simulink model "chap5_5sim"  (Simulink 5.0)
settings: Solver=ode45  StartTime=0.0  StopTime=5.0  FixedStep=0.001  RelTol=1e-3
PreLoadFcn:
  | i=k;
settings Model: LastModifiedBy=Administrator  MaxDataPoints=10000  RTWOptions="-aEnforceIntegerDowncast=1 -aExtMode=0 -aExtModeTesting=0 -aFoldNonRolledExpr=1 -aForceParamTrailComments=0 -aGenerateComments=1 -aGenerateReport=0 -aIgnoreCustomStorageClasses=1 -aIncDataTypeInIds=0 -aIncHierarchyInIds=0 -aInlineInvariantSignals=0 -aInlinedPrmAccess=\"Literals\" -aLocalBlockOutputs=1 -aLogVarNameModifier=\"rt_\" -aMaxRTWIdLen=31 -aPrefixModelToSubsysFcnNames=1 -aRTWVerbose=1 -aRollThreshold=5 -aShowEliminatedStatements=0"

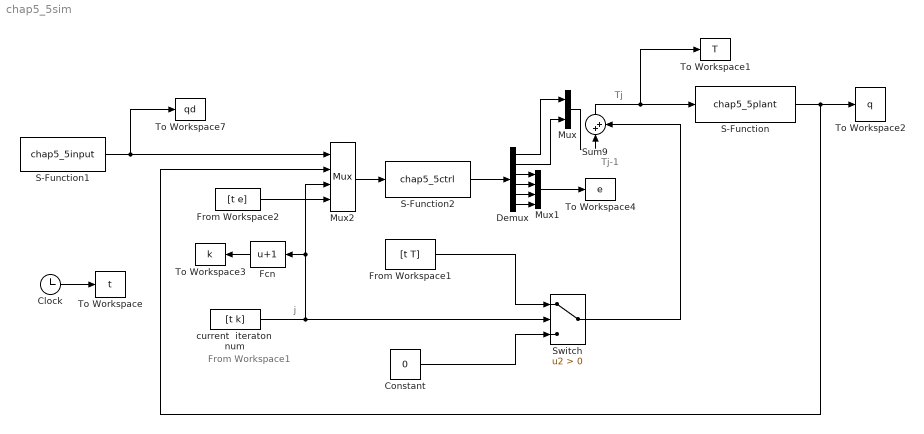
== system chap5_5sim ==
  note: Tj
  note: Tj-1
  note: j
  note: From
      | Workspace1
  Clock : Clock
      settings: Decimation=10
  Constant : Constant  Value=0
  Demux : Demux  Outputs=6
  Fcn : Fcn  Orientation=left  Expr=u+1
  From Workspace1 : FromWorkspace  VariableName=[t T]  SampleTime=0
  From Workspace2 : FromWorkspace  VariableName=[t e]  SampleTime=0
  Mux : Mux  Inputs=2
  Mux1 : Mux
  Mux2 : Mux
  S-Function : S-Function  FunctionName=chap5_5plant
  S-Function1 : S-Function  FunctionName=chap5_5input
  S-Function2 : S-Function  FunctionName=chap5_5ctrl
  Sum9 : Sum  Orientation=up  Inputs=|++  SaturateOnIntegerOverflow=on
  Switch : Switch  Criteria=u2 > Threshold  SaturateOnIntegerOverflow=on
  To Workspace : ToWorkspace  VariableName=t  SampleTime=-1  SaveFormat=Array
  To Workspace1 : ToWorkspace  VariableName=T  SampleTime=-1  SaveFormat=Array
  To Workspace2 : ToWorkspace  VariableName=q  SampleTime=-1  SaveFormat=Array
  To Workspace3 : ToWorkspace  VariableName=k  SampleTime=-1  SaveFormat=Array
  To Workspace4 : ToWorkspace  VariableName=e  SampleTime=-1  SaveFormat=Array
  To Workspace7 : ToWorkspace  VariableName=qd  SampleTime=-1  SaveFormat=Array
  current  iteraton  num : FromWorkspace  VariableName=[t k]  SampleTime=0
  wires:
  S-Function/1 -> To Workspace2/1, Mux2/2
  Clock/1 -> To Workspace/1
  S-Function1/1 -> To Workspace7/1, Mux2/1
  Sum9/1 -> S-Function/1, To Workspace1/1
  Switch/1 -> Sum9/2
  Constant/1 -> Switch/3
  Mux2/1 -> S-Function2/1
  From Workspace1/1 -> Switch/1
  current  iteraton  num/1 -> Switch/2, Fcn/1, Mux2/3
  Fcn/1 -> To Workspace3/1
  Mux/1 -> Sum9/1
  S-Function2/1 -> Demux/1
  Demux/1 -> Mux/1
  Demux/2 -> Mux/2
  Demux/3 -> Mux1/1
  Demux/5 -> Mux1/3
  Demux/4 -> Mux1/2
  Demux/6 -> Mux1/4
  Mux1/1 -> To Workspace4/1
  From Workspace2/1 -> Mux2/4
